simulink model "reciever"  (R2022a)
settings: Solver=FixedStepAuto  StartTime=0.0  StopTime=10.0  RelTol=1e-3
libraries: androidcommunicationlib x5, androiduilib x3, androidaudiovideolib x2
settings Model: Creator=GautamVashishtha  LastModifiedBy=GautamVashishtha
settings OptimizationCC: EnhancedBackFolding=on  PassReuseOutputArgsAs=Individual arguments  ZeroExternalMemoryAtStartup=off  ZeroInternalMemoryAtStartup=off  MaxStackSize=64  OptimizeBlockOrder=speed  DifferentSizesBufferReuse=on  OptimizationCustomize=off  EfficientTunableParamExpr=on
settings DebuggingCC: ParameterTunabilityLossMsg=error
settings HardwareCC: ProdBitPerPointer=32  ProdBitPerSizeT=32  ProdBitPerPtrDiffT=32  ProdLargestAtomicInteger=Long  ProdLargestAtomicFloat=Double  ProdWordSize=32  ProdHWDeviceType=ARM Compatible->ARM Cortex  UseEmbeddedCoderFeatures=off  UseSimulinkCoderFeatures=off
settings SFSimCC: MATLABDynamicMemAlloc=off
settings RTWCC: SystemTargetFile=ert.tlc  HardwareBoard=Android Device  TLCOptions="-aInlineSetEventsForThisBaseRateFcn=TLC_FALSE -aSuppressMultiTaskScheduler=TLC_FALSE  -aRateBasedStepFcn=0"  TemplateMakefile=ert_default_tmf  RTWVerbose=off  Toolchain=Android SDK/NDK Tools
settings CodeAppCC: ForceParamTrailComments=on  IgnoreCustomStorageClasses=off  OperatorAnnotations=on  SimulinkDataObjDesc=on  SFDataObjDesc=on  InsertBlockDesc=on
settings ERTTargetCC: SupportNonInlinedSFcns=on

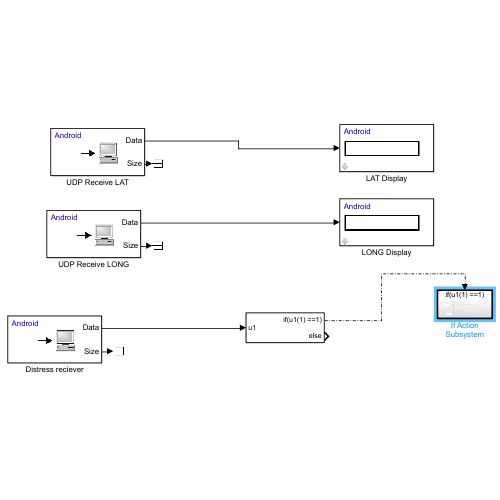
[thumbnail: Simulink's stored preview of the top-level diagram]
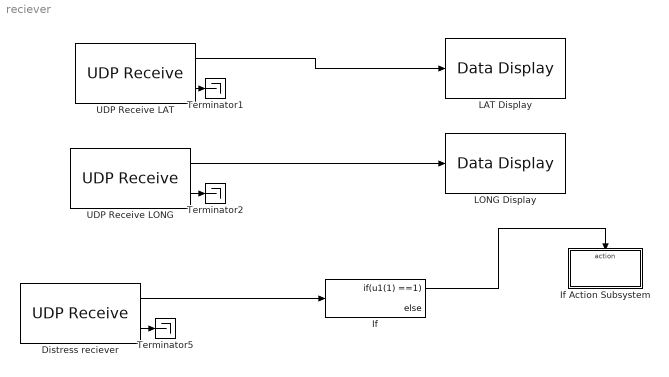
== system reciever ==
  Distress reciever : androidcommunicationlib/UDP Receive  localURL='0.0.0.0'  localPort=3000  remoteURL='0.0.0.0'  remotePort=-1  recvBufferSize=8192  signalDatatype=double  dims=255  isVarSize=off  showBlockingTime=off  blockingTime=0  sampletime=0.0002040816326530612  blockPlatform=Android
      settings: SourceProductBaseCode=ANDROID
  If : If  IfExpression=u1(1) ==1
  If Action Subsystem : Subsystem  TreatAsAtomicUnit=on
  LAT Display : androiduilib/Data Display  DataDisplayId=reciever/Data_Display  Format=Float  Precision=6  SimulateUsing=Code generation  blockPlatform=Android
      settings: SourceProductBaseCode=ANDROID
  LONG Display : androiduilib/Data Display  DataDisplayId=reciever/Data_Display  Format=Float  Precision=6  SimulateUsing=Code generation  blockPlatform=Android
      settings: SourceProductBaseCode=ANDROID
  Terminator1 : Terminator
  Terminator2 : Terminator
  Terminator5 : Terminator
  UDP Receive LAT : androidcommunicationlib/UDP Receive  localURL='0.0.0.0'  localPort=5000  remoteURL='0.0.0.0'  remotePort=-1  recvBufferSize=8192  signalDatatype=double  dims=255  isVarSize=off  showBlockingTime=off  blockingTime=0  sampletime=0.1  blockPlatform=Android
      settings: SourceProductBaseCode=ANDROID
  UDP Receive LONG : androidcommunicationlib/UDP Receive  localURL='0.0.0.0'  localPort=4000  remoteURL='0.0.0.0'  remotePort=-1  recvBufferSize=8192  signalDatatype=double  dims=255  isVarSize=off  showBlockingTime=off  blockingTime=0  sampletime=0.1  blockPlatform=Android
      settings: SourceProductBaseCode=ANDROID
  wires:
  Distress reciever/2 -> Terminator5/1
  Distress reciever/1 -> If/1
  If/1 -> If Action Subsystem/Action
  UDP Receive LAT/2 -> Terminator1/1
  UDP Receive LONG/2 -> Terminator2/1
  UDP Receive LAT/1 -> LAT Display/1
  UDP Receive LONG/1 -> LONG Display/1

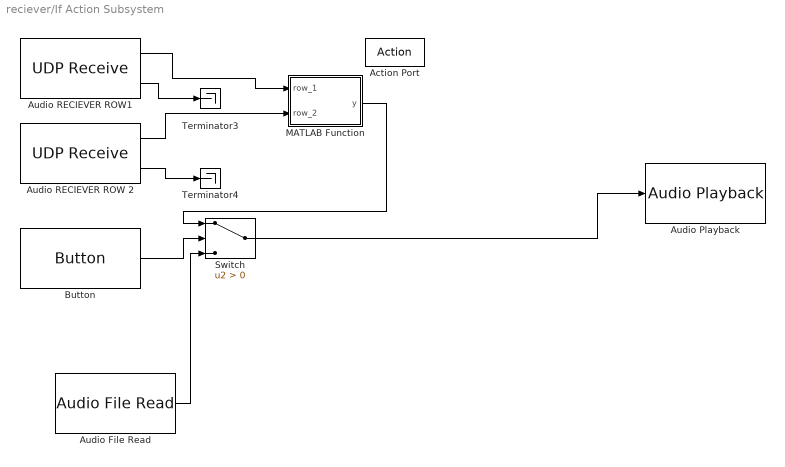
== system reciever/If Action Subsystem ==
  Action Port : ActionPort  ActionPortLabel=if(u1(1) ==1)
  Audio File Read : androidaudiovideolib/Audio File Read  FileName=C:\work\sem_7\DSP\Assignment_matlab\who-let-the-dogs-out-ringtone.mp3  FrameSize=9
      settings: SourceProductBaseCode=ANDROID
  Audio Playback : androidaudiovideolib/Audio Playback  SampleFreq=16000  AudioSamplingFreq=16000  SampleTime=0.1  DeviceStr=0  QueueDuration=0  BlockPlatform=Android
      settings: SourceProductBaseCode=ANDROID
  Audio RECIEVER ROW 2 : androidcommunicationlib/UDP Receive  localURL='0.0.0.0'  localPort=8000  remoteURL='0.0.0.0'  remotePort=-1  recvBufferSize=8192  signalDatatype=int16  dims=4410  isVarSize=off  showBlockingTime=off  blockingTime=0  sampletime=0.01  blockPlatform=Android
      settings: SourceProductBaseCode=ANDROID
  Audio RECIEVER ROW1 : androidcommunicationlib/UDP Receive  localURL='0.0.0.0'  localPort=6000  remoteURL='0.0.0.0'  remotePort=-1  recvBufferSize=8192  signalDatatype=int16  dims=4410  isVarSize=off  showBlockingTime=off  blockingTime=0  sampletime=0.01  blockPlatform=Android
      settings: SourceProductBaseCode=ANDROID
  Button : androiduilib/Button  ButtonState=Not pressed  State=off  SampleTime=0.1  BlockPlatform=Android
      settings: SourceProductBaseCode=ANDROID
  MATLAB Function : MATLAB Function  TreatAsAtomicUnit=on
  Switch : Switch  Criteria=u2 > Threshold  SaturateOnIntegerOverflow=off  InputSameDT=off
  Terminator3 : Terminator
  Terminator4 : Terminator
  wires:
  Audio RECIEVER ROW1/2 -> Terminator3/1
  Audio RECIEVER ROW1/1 -> MATLAB Function/1(row_1)
  Audio RECIEVER ROW 2/2 -> Terminator4/1
  Audio RECIEVER ROW 2/1 -> MATLAB Function/2(row_2)
  Button/1 -> Switch/2
  MATLAB Function/1(y) -> Switch/1
  Audio File Read/1 -> Switch/3
  Switch/1 -> Audio Playback/1

== matlab function reciever/If Action Subsystem/MATLAB Function ==
  data: row_1 input; y output; row_2 input
function y = fcn(row_1,row_2)

y = [row_1,row_2];
